simulink library "gyroscope_lib"  (R2018b)
settings: Solver=VariableStepAuto  StartTime=0.0  StopTime=10.0  RelTol=1e-3
undefined symbols (not defined in the file): DiscIntNeverNeededParam, simParams
libraries: simulink x3
settings Model: Creator=colem  LastModifiedBy=taylorreynolds

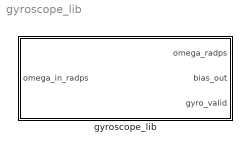
== system gyroscope_lib ==
  gyroscope_lib : Subsystem  mask{id_s=1}
      mask prompts: id_s "Choose the sensor ID"
      mask TypeOptions id_s: 1 | 2 | 3
      mask DialogControl DescTextVar Prompt: SOCi gyroscope model. The spacecraft has three Bosch BMI055 gyroscopes.

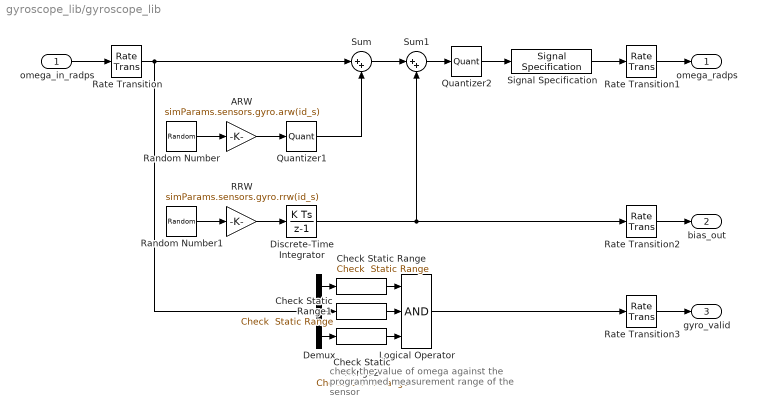
== system gyroscope_lib/gyroscope_lib ==
  note: check the value of omega against
      | the programmed measurement range
      | of the sensor
  omega_in_radps : Inport
  ARW : Gain  Gain=simParams.sensors.gyro.arw(id_s)
  Check Static Range : simulink/Model Verification/Check  Static Range  Description=simParams.sensors.gyro.w_min(id_s) <= u <= simParams.sensors.gyro.w_max(id_s)  max=simParams.sensors.gyro.w_max(id_s)  max_included=on  min=simParams.sensors.gyro.w_min(id_s)  min_included=on  enabled=on  stopWhenAssertionFail=off  export=on  icon=graphic
      settings: SourceProductName=Simulink  SourceProductBaseCode=SL
  Check Static Range1 : simulink/Model Verification/Check  Static Range  Description=simParams.sensors.gyro.w_min(id_s) <= u <= simParams.sensors.gyro.w_max(id_s)  max=simParams.sensors.gyro.w_max(id_s)  max_included=on  min=simParams.sensors.gyro.w_min(id_s)  min_included=on  enabled=on  stopWhenAssertionFail=off  export=on  icon=graphic
      settings: SourceProductName=Simulink  SourceProductBaseCode=SL
  Check Static Range2 : simulink/Model Verification/Check  Static Range  Description=simParams.sensors.gyro.w_min(id_s) <= u <= simParams.sensors.gyro.w_max(id_s)  max=simParams.sensors.gyro.w_max(id_s)  max_included=on  min=simParams.sensors.gyro.w_min(id_s)  min_included=on  enabled=on  stopWhenAssertionFail=off  export=on  icon=graphic
      settings: SourceProductName=Simulink  SourceProductBaseCode=SL
  Demux : Demux  Outputs=3
  Discrete-Time Integrator : DiscreteIntegrator  InitialCondition=simParams.sensors.gyro.bias_init(id_s)  SampleTime=-1  ICPrevOutput=DiscIntNeverNeededParam  ICPrevScaledInput=DiscIntNeverNeededParam
  Logical Operator : Logic  Inputs=3  AllPortsSameDT=off  OutDataTypeStr=boolean
  Quantizer1 : Quantizer  QuantizationInterval=simParams.sensors.gyro.resolution(id_s)
  Quantizer2 : Quantizer  QuantizationInterval=simParams.sensors.gyro.resolution(id_s)
  RRW : Gain  Gain=simParams.sensors.gyro.rrw(id_s)
  Random Number : RandomNumber  Mean=[0 0 0]  Variance=[1 1 1]  Seed=simParams.sensors.gyro.seed_arw(:,id_s)  SampleTime=simParams.sensors.gyro.sample_time_s
  Random Number1 : RandomNumber  Mean=[0 0 0]  Variance=[1 1 1]  Seed=simParams.sensors.gyro.seed_rrw(:,id_s)  SampleTime=simParams.sensors.gyro.sample_time_s
  Rate Transition : RateTransition  InitialCondition=simParams.initialConditions.w0  OutPortSampleTime=simParams.sensors.gyro.sample_time_s
  Rate Transition1 : RateTransition  InitialCondition=simParams.initialConditions.w0
  Rate Transition2 : RateTransition  InitialCondition=simParams.sensors.gyro.bias_init(id_s)
  Rate Transition3 : RateTransition  InitialCondition=1
  Signal Specification : SignalSpecification  Dimensions=3
  Sum : Sum  Inputs=|++
  Sum1 : Sum  Inputs=|++
  omega_radps : Outport
  bias_out : Outport  Port=2
  gyro_valid : Outport  Port=3
  wires:
  Random Number/1 -> ARW/1
  Random Number1/1 -> RRW/1
  ARW/1 -> Quantizer1/1
  omega_in_radps/1 -> Rate Transition/1
  Sum/1 -> Sum1/1
  RRW/1 -> Discrete-Time Integrator/1
  Logical Operator/1 -> Rate Transition3/1
  Discrete-Time Integrator/1 -> Rate Transition2/1, Sum1/2
  Quantizer1/1 -> Sum/2
  Sum1/1 -> Quantizer2/1
  Quantizer2/1 -> Signal Specification/1
  Rate Transition/1 -> Demux/1, Sum/1
  Rate Transition1/1 -> omega_radps/1
  Rate Transition2/1 -> bias_out/1
  Rate Transition3/1 -> gyro_valid/1
  Demux/3 -> Check Static Range2/1
  Demux/2 -> Check Static Range1/1
  Demux/1 -> Check Static Range/1
  Check Static Range1/1 -> Logical Operator/2
  Check Static Range/1 -> Logical Operator/1
  Check Static Range2/1 -> Logical Operator/3
  Signal Specification/1 -> Rate Transition1/1
